simulink model "Continuous_Two_Input_Events_2018a"  (R2018a)
settings: Solver=VariableStepAuto  StartTime=0.0  StopTime=40  RelTol=1e-3
settings Model: Creator=apple  LastModifiedBy=BEAR
settings DataIOCC: ReturnWorkspaceOutputs=on
settings SFSimCC: SimUseLocalCustomCode=on
settings RTWCC: RTWUseLocalCustomCode=on

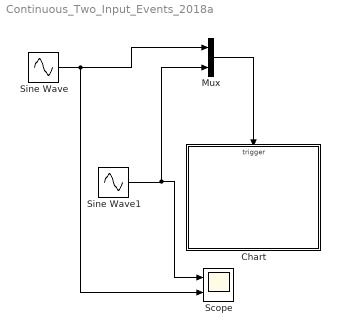
== system Continuous_Two_Input_Events_2018a ==
  Chart : Stateflow chart  TreatAsAtomicUnit=on
  Mux : Mux  Inputs=2
  Scope : Scope  NumInputPorts=2
  Sine Wave : Sin  SampleTime=0
  Sine Wave1 : Sin  Phase=1  SampleTime=0
  wires:
  Sine Wave1/1 -> Mux/2, Scope/1
  Sine Wave/1 -> Scope/2, Mux/1
  Mux/1 -> Chart/Trigger

== stateflow chart Continuous_Two_Input_Events_2018a/Chart ==
  settings: executeAtInitialization=1
  state On
    en:f("Entry_On");
    du:f("During_On");
    ex:f("Exit_On");
    On -> On [order 1] : E_one/{f("E1_on")}
  state Off
    en:f("Entry_Off");
    du:f("During_Off");
    ex:f("Exit_Off");
    Off -> Off [order 1] : E_two/{f("E2_off")}
  (default) -> On
  On -> Off [order 1] : E_two/{f("E2")}
  Off -> On [order 1] : E_one/{f("E1")}
  data: s function_input
  events: E_one input RISING_EDGE_EVENT; E_two input RISING_EDGE_EVENT
  function f(s):
    | function f(s)
    |   fprintf(s+"\n");
